simulink model "PI7s"  (R2015a)
settings: Solver=ode45  StartTime=0.0  StopTime=1  RelTol=1e-3
libraries: simulink x1
settings Model: Creator=Edsilvio  LastModifiedBy=Tuor

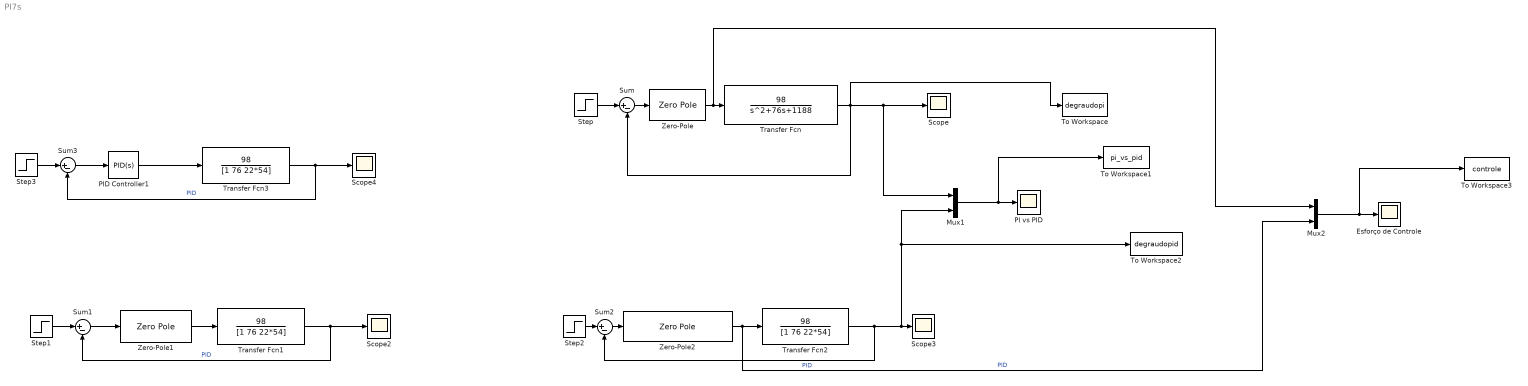
== system PI7s ==
  Esforço de Controle : Scope
      settings: YMin=-1  YMax=1.24  SaveName=ScopeData5
  Mux1 : Mux  Inputs=2
  Mux2 : Mux  Inputs=2
  PI vs PID : Scope
      settings: YMin=-1  YMax=1.24
  PID Controller1 : simulink/Continuous/PID Controller  Controller=PID  TimeDomain=Continuous-time  SampleTime=-1  IntegratorMethod=Forward Euler  FilterMethod=Forward Euler  Form=Ideal  UseFilter=on  ControllerParametersSource=internal  P=96.807280123132  I=19.532770932661  D=0.0115522224772921  N=13658.0621164575  InitialConditionSource=internal  InitialConditionForIntegrator=0  InitialConditionForFilter=0  ExternalReset=none  LimitOutput=off  UpperSaturationLimit=inf  LowerSaturationLimit=-inf  LinearizeAsGain=on  AntiWindupMode=none  Kb=1  TrackingMode=off  Kt=1  PParamMin=[]  PParamMax=[]  IParamMin=[]  IParamMax=[]  DParamMin=[]  DParamMax=[]  NParamMin=[]  NParamMax=[]  KbParamMin=[]  KbParamMax=[]  KtParamMin=[]  KtParamMax=[]  POutMin=[]  POutMax=[]  IOutMin=[]  IOutMax=[]  DOutMin=[]  DOutMax=[]  NOutMin=[]  NOutMax=[]  KbOutMin=[]  KbOutMax=[]  KtOutMin=[]  KtOutMax=[]  IntegratorOutMin=[]  IntegratorOutMax=[]  FilterOutMin=[]  FilterOutMax=[]  SumOutMin=[]  SumOutMax=[]  SumI1OutMin=[]  SumI1OutMax=[]  SumI2OutMin=[]  SumI2OutMax=[]  SumI3OutMin=[]  SumI3OutMax=[]  SumDOutMin=[]  SumDOutMax=[]  SaturationOutMin=[]  SaturationOutMax=[]  IntegratorContinuousStateAttributes=''  IntegratorStateMustResolveToSignalObject=off  IntegratorRTWStateStorageClass=Auto  FilterContinuousStateAttributes=''  FilterStateMustResolveToSignalObject=off  FilterRTWStateStorageClass=Auto  DifferentiatorICPrevScaledInput=0  DifferentiatorOutMin=[]  DifferentiatorOutMax=[]
  Scope{,2..4} (4 alike) : Scope
      Scope settings: YMin=-1  YMax=1.24
      Scope2 settings: YMin=-1  YMax=1  SaveName=ScopeData2
      Scope3 settings: YMin=-1  YMax=1.4  SaveName=ScopeData3
      Scope4 settings: YMin=-1  YMax=1.4  SaveName=ScopeData4
  Step{,1..3} (4 alike) : Step  Time=0  SampleTime=0
  Sum{,1..3} (4 alike) : Sum  Inputs=|+-
  To Workspace : ToWorkspace  VariableName=degraudopi  SaveFormat=Timeseries  SampleTime=-1
  To Workspace1 : ToWorkspace  VariableName=pi_vs_pid  SaveFormat=Timeseries  SampleTime=-1
  To Workspace2 : ToWorkspace  VariableName=degraudopid  SaveFormat=Timeseries  SampleTime=-1
  To Workspace3 : ToWorkspace  VariableName=controle  SaveFormat=Timeseries  SampleTime=-1
  Transfer Fcn : TransferFcn  Numerator=98  Denominator=[1 76 1188]
  Transfer Fcn1 : TransferFcn  Numerator=98  Denominator=[1 76 22*54]
  Transfer Fcn2 : TransferFcn  Numerator=98  Denominator=[1 76 22*54]
  Transfer Fcn3 : TransferFcn  Numerator=98  Denominator=[1 76 22*54]
  Zero-Pole : ZeroPole  Zeros=[-24.2]  Poles=[0]  Gain=12
  Zero-Pole1 : ZeroPole  Zeros=[-48.6 -24.2]  Poles=[-87 0]  Gain=33.7
  Zero-Pole2 : ZeroPole  Zeros=[-24.2 -59.4]  Poles=[-200 0]  Gain=95.32
  wires:
  Step/1 -> Sum/1
  Sum/1 -> Zero-Pole/1
  Transfer Fcn/1 -> Sum/2, Mux1/1, Scope/1, To Workspace/1
  Step2/1 -> Sum2/1
  Sum2/1 -> Zero-Pole2/1
  Transfer Fcn2/1 -> Mux1/2, To Workspace2/1, Scope3/1, Sum2/2  "PID"
  Mux1/1 -> To Workspace1/1, PI vs PID/1
  Step1/1 -> Sum1/1
  Sum1/1 -> Zero-Pole1/1
  Transfer Fcn1/1 -> Sum1/2, Scope2/1  "PID"
  Zero-Pole1/1 -> Transfer Fcn1/1
  Step3/1 -> Sum3/1
  Sum3/1 -> PID Controller1/1
  Transfer Fcn3/1 -> Sum3/2, Scope4/1  "PID"
  PID Controller1/1 -> Transfer Fcn3/1
  Zero-Pole/1 -> Mux2/1, Transfer Fcn/1
  Zero-Pole2/1 -> Mux2/2, Transfer Fcn2/1  "PID"
  Mux2/1 -> To Workspace3/1, Esforço de Controle/1
